simulink model "dp2"  (R2017a)
settings: Solver=FixedStepDiscrete  StartTime=0.0  StopTime=20  FixedStep=1.0  RelTol=1e-3
InitFcn:
  | xs = 0:0.1:1;
  | us = 0:0.2:1;
  | [ugrid,xgrid] = meshgrid(us,xs);
undefined symbols (not defined in the file): magnitude, ugrid, xgrid
libraries: simulink x1
settings Model: Creator=thomas  LastModifiedBy=thomas

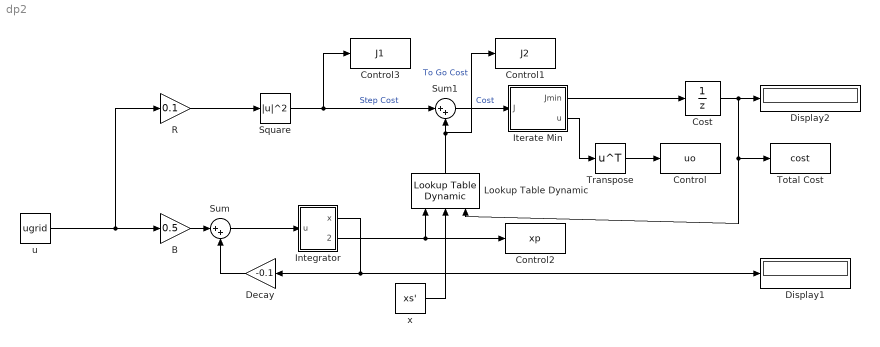
== system dp2 ==
  B : Gain  Gain=0.5
  Control : ToWorkspace  VariableName=uo  SampleTime=-1
      settings: Save2DSignal=2-D array (concatenate along first dimension)
  Control1 : ToWorkspace  VariableName=J2  SampleTime=-1
  Control2 : ToWorkspace  VariableName=xp  SampleTime=-1
  Control3 : ToWorkspace  VariableName=J1  SampleTime=-1
  Cost : UnitDelay  InitialCondition=(1-xs)'
  Decay : Gain  Gain=-0.1
  Display1 : Display
  Display2 : Display
  Integrator : Subsystem
  Iterate Min : Subsystem  TreatAsAtomicUnit=on
  Lookup Table Dynamic : simulink/Lookup Tables/Lookup Table Dynamic  LookUpMeth=Interpolation-Use End Values  OutDataType=fixdt('double')  OutScaling=[]  OutputDataTypeScalingMode=Specify via dialog  OutDataTypeStr=double  DoSatur=off
      settings: SourceProductName=Simulink
  R : Gain  Gain=0.1
  Square : Math  Operator=magnitude^2  SaturateOnIntegerOverflow=on
  Sum : Sum  Inputs=|++
  Sum1 : Sum  Inputs=|++
  Total Cost : ToWorkspace  VariableName=cost  SampleTime=-1
      settings: MaxDataPoints=1
  Transpose : Math  Operator=transpose  SaturateOnIntegerOverflow=on
  u : Constant  Value=ugrid  VectorParams1D=off
  x : Constant  Value=xs'  VectorParams1D=off
  wires:
  B/1 -> Sum/1
  R/1 -> Square/1
  u/1 -> B/1, R/1
  Square/1 -> Control3/1, Sum1/1  "Step Cost"
  Decay/1 -> Sum/2
  Cost/1 -> Total Cost/1, Lookup Table Dynamic/3, Display2/1
  Lookup Table Dynamic/1 -> Control1/1, Sum1/2  "To Go Cost"
  Integrator/1(x) -> Display1/1, Decay/1
  Sum/1 -> Integrator/1(u)
  Integrator/2(x+) -> Control2/1, Lookup Table Dynamic/1
  Sum1/1 -> Iterate Min/1(J)  "Cost"
  Iterate Min/1(Jmin) -> Cost/1
  x/1 -> Lookup Table Dynamic/2
  Iterate Min/2(u) -> Transpose/1
  Transpose/1 -> Control/1

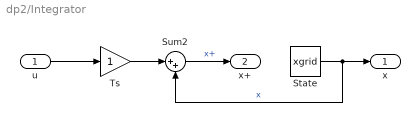
== system dp2/Integrator ==
  u : Inport
  State : Constant  Value=xgrid  VectorParams1D=off
  Sum2 : Sum  Inputs=|++
  Ts : Gain
  x : Outport
  x+ : Outport  Port=2
  wires:
  u/1 -> Ts/1
  Ts/1 -> Sum2/1
  Sum2/1 -> x+/1  "x+"
  State/1 -> x/1, Sum2/2  "x"

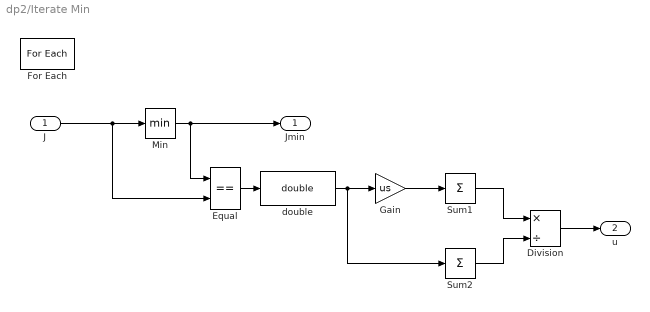
== system dp2/Iterate Min ==
  J : Inport  Partition=on  PartitionDimension=1  PartitionWidth=1
  Division : Product  Inputs=*/
  Equal : RelationalOperator  Operator===  OutDataTypeStr=boolean  ZeroCross=off  RndMeth=Simplest
  For Each : ForEach  DisableCoverage=on  IndexMode=One-based
  Gain : Gain  Gain=us
  Min : MinMax
  Sum1 : Sum  Inputs=+  CollapseMode=Specified dimension  CollapseDim=2
  Sum2 : Sum  Inputs=+  CollapseMode=Specified dimension  CollapseDim=2
  double : DataTypeConversion  OutDataTypeStr=double
  Jmin : Outport  ConcatenationDimension=1
  u : Outport  Port=2  ConcatenationDimension=1
  wires:
  J/1 -> Equal/2, Min/1
  Min/1 -> Jmin/1, Equal/1
  Equal/1 -> double/1
  Gain/1 -> Sum1/1
  Division/1 -> u/1
  Sum1/1 -> Division/1
  Sum2/1 -> Division/2
  double/1 -> Sum2/1, Gain/1
